simulink library "Library_ASK"  (R2018b)
settings: Solver=VariableStepAuto  StartTime=0.0  StopTime=10.0  RelTol=1e-3  EnableMultiTasking=on
undefined symbols (not defined in the file): akt_2GTR_az_HA, akt_2GTR_az_VA, akt_2GTR_rn_HA, akt_2GTR_rn_VA, akt_GTR_az_HA, akt_GTR_az_VA, akt_GTR_rn_HA, akt_GTR_rn_VA, alpha, b_zahn, beta_b, breakpointset, choose_ulg, DiscIntNeverNeededParam, eps_1, eps_2, eps_alpha, eta_aa, eta_Kegel_max, Fx_LSD_max, Fx_mUELG_max, i_DF, i_Kegelrad_OD, i_TRM_G1_HA, i_TRM_G1_VA, i_TRM_G2_HA, i_TRM_G2_VA, i_TRM_HA, i_TRM_Stufe_1_HA, i_TRM_Stufe_1_VA, i_TRM_Stufe_2_HA, i_TRM_Stufe_2_VA, i_TRM_VA, M_Cl_LSD_max, M_Cl_mUELG_max, M_EM_max, M_Kupplung_mUELG_Schlepp, mu_cl_LSD, mu_cl_mUELG, n_EM_max, n_Stufen_TRM_HA, n_Stufen_TRM_VA, ndyn_oil, nreib_LSD, nreib_mUELG, par_MDT, par_VEH, Ra, rm_LSD, rm_mUELG, select_Traktion_split, stepsize, wkg_Diff_mUELG, wkg_GTR, X_L, z_atts, z_ayc, z_ayc_lr, z_ayc_rl
libraries: simulink x23, $bdroot x6
(part 1 of 4)
settings Model: Creator=ga25fis  LastModifiedBy=ga35gug
settings DataIOCC: LimitDataPoints=on
settings OptimizationCC: LifeSpan=inf
settings DebuggingCC: AllowSymbolicDim=off  SFUnexpectedBacktrackingDiag=warning  SFNoUnconditionalDefaultTransitionDiag=warning  SFExecutionAtInitializationDiag=none
settings ModelReferenceCC: PropagateSignalLabelsOutOfModel=off
settings SFSimCC: SimUseLocalCustomCode=off
settings RTWCC: RTWUseLocalCustomCode=off
settings CodeAppCC: StateflowObjectComments=on
settings GRTTargetCC: TargetLangStandard=C89/C90 (ANSI)
settings ConfigComp: CovMetricSettings=dw  CovHtmlReporting=on  CovSaveCumulativeToWorkspaceVar=on  CovSaveSingleToWorkspaceVar=on  CovExternalEMLEnable=off

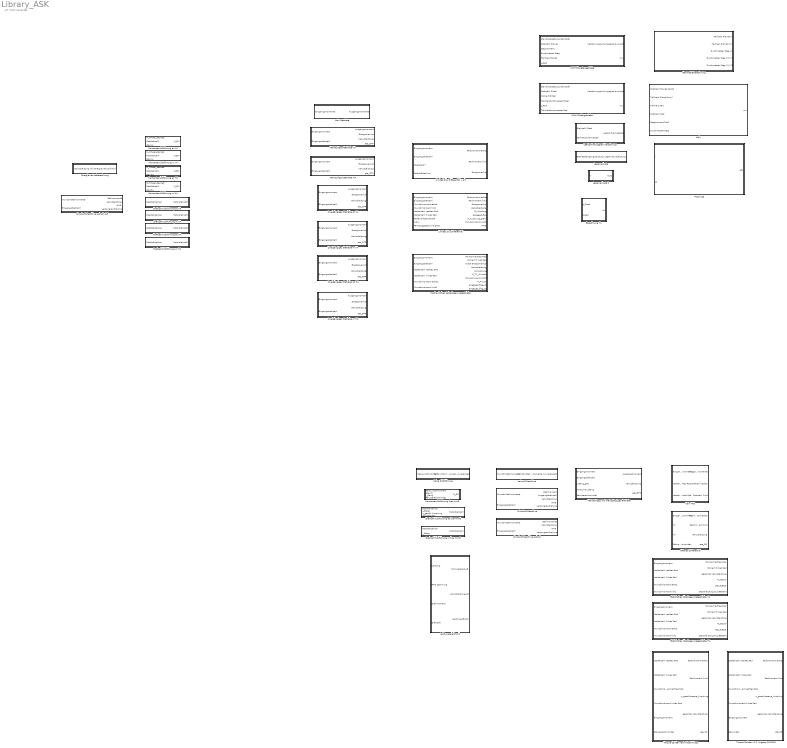
== system Library_ASK ==
  note: ALT / Nicht verwendet
  Berechnung Hv : Subsystem
  Drehzahlrückführung az HA : Subsystem
      mask Display: set_param(gcb, 'BackgroundColor', '[0.9,0.7,1]');
  Drehzahlrückführung az VA : Subsystem
      mask Display: set_param(gcb, 'BackgroundColor', '[0.9,0.7,1]');
  Drehzahlrückführung az fuer mmG : Subsystem
      mask Display: set_param(gcb, 'BackgroundColor', '[0.9,0.7,1]');
  Drehzahlrückführung rn HA : Subsystem
      mask Display: set_param(gcb, 'BackgroundColor', '[0.9,0.7,1]');
  Drehzahlrückführung rn VA : Subsystem
      mask Display: set_param(gcb, 'BackgroundColor', '[0.9,0.7,1]');
  Drehzahlrückführung rn fuer mmG : Subsystem
      mask Display: set_param(gcb, 'BackgroundColor', '[0.9,0.7,1]');
  Elektrisches Überlagerungsgetriebe HA : Subsystem
      settings: MinAlgLoopOccurrences=on
      mask Display: set_param(gcb, 'BackgroundColor', '[0,1,0.6]');
  Elektrisches Überlagerungsgetriebe VA : Subsystem
      settings: MinAlgLoopOccurrences=on
      mask Display: set_param(gcb, 'BackgroundColor', '[0,1,0.6]');
  Energieverlustberechnung : Subsystem
      mask Display: set_param(gcb, 'BackgroundColor', '[0.3,0.3,0.6]');
  Geometrieberechnung : Subsystem
  Kein Getriebe : Subsystem
      settings: MinAlgLoopOccurrences=on
      mask Display: set_param(gcb, 'BackgroundColor', '[0.9,0.1,0.4]');
  Kein MVS : Subsystem
      mask Display: set_param(gcb, 'BackgroundColor', '[0,1,0.6]');
  Keine E-Maschine : Subsystem
      settings: MinAlgLoopOccurrences=on
      mask Display: set_param(gcb, 'BackgroundColor', '[0.5,0.7,1]');
  Keine Rückführung : Subsystem
      mask Display: set_param(gcb, 'BackgroundColor', '[0.9,0.7,1]');
  Kelly : Subsystem
  Lagerverluste : Subsystem
  Lagerverluste 2 : Subsystem
  Leerlaufverlustgrad Verzahnung : Subsystem
  Leistungselektronik : Subsystem  mask{Efficiency_Map=0, Current=0, Voltage=0, Powerfactor=0, Powerfactor_Map=0, Torque=0, Speed=0}
      mask prompts: Current "Strom"; Voltage "Spannung"; Torque "Drehmoment"; Speed "Drehzahl"
      mask DialogControl ParameterGroupVar Prompt: Efficiency_Map
      mask DialogControl ParameterGroupVar_copy Prompt: Powerfactor_Map
  Limited Slip Differential : Subsystem
      settings: MinAlgLoopOccurrences=on
      mask Display: set_param(gcb, 'BackgroundColor', '[0,1,0.6]');
  "Limited Slip Differential -- alt" : Subsystem
      settings: MinAlgLoopOccurrences=on
      mask Display: set_param(gcb, 'BackgroundColor', '[0,1,0.6]');
  Mehrstufiges Getriebe HA : Subsystem
      settings: MinAlgLoopOccurrences=on
      mask Display: set_param(gcb, 'BackgroundColor', '[0.9,0.1,0.4]');
  Mehrstufiges Getriebe VA : Subsystem
      settings: MinAlgLoopOccurrences=on
      mask Display: set_param(gcb, 'BackgroundColor', '[0.9,0.1,0.4]');
  Mehrstufiges und mehrgängiges Getriebe : Subsystem
      settings: MinAlgLoopOccurrences=on
      mask Display: set_param(gcb, 'BackgroundColor', '[0.9,0.1,0.4]');
  Momentenrückführung az HA : Subsystem
      mask Display: set_param(gcb, 'BackgroundColor', '[0.9,0.7,1]');
  Momentenrückführung az VA : Subsystem
      mask Display: set_param(gcb, 'BackgroundColor', '[0.9,0.7,1]');
  Momentenrückführung fuer mmG : Subsystem
      mask Display: set_param(gcb, 'BackgroundColor', '[0.9,0.7,1]');
  Momentenrückführung rn HA : Subsystem
      mask Display: set_param(gcb, 'BackgroundColor', '[0.9,0.7,1]');
  Momentenrückführung rn VA : Subsystem
      mask Display: set_param(gcb, 'BackgroundColor', '[0.9,0.7,1]');
  NWH Planetengetriebe : Subsystem
      mask Display: set_param(gcb, 'BackgroundColor', '[0.8,0.8,0.8]');
  NWH Stufengetriebe : Subsystem
      mask Display: set_param(gcb, 'BackgroundColor', '[0.8,0.8,0.8]');
  Offenes Differential : Subsystem  mask{M_max=par_MDT.VA.em.M_max_mot, i_max=par_MDT.VA.trans.imax}
      settings: MinAlgLoopOccurrences=on
      mask Display: set_param(gcb, 'BackgroundColor', '[0,1,0.6]');
  Poppinga : Subsystem
  Simple E-Maschine : Subsystem  mask{Mot_Mmax_Curve=par_MDT.VA.em.MaxMotorTrqCurve_M, Mot_nmax_Curve=par_MDT.VA.em.MaxMotorTrqCurve_w, Gen_Mmax_Curve=par_MDT.VA.em.MaxGeneratorTrqCurve_M, Gen_nmax_Curve=par_MDT.VA.em.MaxGeneratorTrqCurve_w, Mot_Pesce_Mat=par_MDT.VA.em.MotorEffMap3D, Mot_Pesce_y=par_MDT.VA.em.MotorEffMap3D_w, Mot_Pesce_z=par_MDT.VA.em.MotorEffMap3D_M, Gen_Pesce_Mat=par_MDT.VA.em.GeneratorEffMap3D, Gen_Pesce_y=par_MDT.VA.em.GeneratorEffMap3D_w, Gen_Pesce_z=par_MDT.VA.em.GeneratorEffMap3D_M}
      settings: MinAlgLoopOccurrences=on
      mask Display: set_param(gcb, 'BackgroundColor', '[0.5,0.7,1]');
  Simple E-Maschine radnah : Subsystem  mask{Mot_Mmax_Curve=par_MDT.VA.em.MaxMotorTrqCurve_M, Mot_nmax_Curve=par_MDT.VA.em.MaxMotorTrqCurve_w, Gen_Mmax_Curve=par_MDT.VA.em.MaxGeneratorTrqCurve_M, Gen_nmax_Curve=par_MDT.VA.em.MaxGeneratorTrqCurve_w, Mot_Pesce_Mat=par_MDT.VA.em.MotorEffMap3D, Mot_Pesce_y=par_MDT.VA.em.MotorEffMap3D_w, Mot_Pesce_z=par_MDT.VA.em.MotorEffMap3D_M, Gen_Pesce_Mat=par_MDT.VA.em.GeneratorEffMap3D, Gen_Pesce_y=par_MDT.VA.em.GeneratorEffMap3D_w, Gen_Pesce_z=par_MDT.VA.em.GeneratorEffMap3D_M}
      settings: MinAlgLoopOccurrences=on
      mask Display: set_param(gcb, 'BackgroundColor', '[0.5,0.7,1]');
  Simple E-Maschine radnah ALT : Subsystem  mask{Mot_Mmax_Curve=par_VEH.dt.em.MmaxCurve_mot_VA, Mot_nmax_Curve=par_VEH.dt.em.nmaxCurve_mot_VA, Gen_Mmax_Curve=par_VEH.dt.em.MmaxCurve_gen_VA, Gen_nmax_Curve=par_VEH.dt.em.nmaxCurve_gen_VA, Mot_Pesce_Mat=par_VEH.dt.em.EffMapData_mot_VA, Mot_Pesce_y=par_VEH.dt.em.MotorEffMap3D_y_VA, Mot_Pesce_z=par_VEH.dt.em.MotorEffMap3D_z_VA, Gen_Pesce_Mat=par_VEH.dt.em.EffMapData_gen_VA, Gen_Pesce_y=par_VEH.dt.em.GeneratorEffMap3D_y_VA, Gen_Pesce_z=par_VEH.dt.em.GeneratorEffMap3D_z_VA}
      settings: MinAlgLoopOccurrences=on
      mask Display: set_param(gcb, 'BackgroundColor', '[0.5,0.7,1]');
  Torque Splitter nach Arbeit Tripps : Subsystem  TreatAsAtomicUnit=on
  Torque Splitter v2 C. Angerer 10/2018 : Subsystem
  Zweigängiges Getriebe az HA : Subsystem
      mask Display: set_param(gcb, 'BackgroundColor', '[0.9,0.1,0.4]');
  Zweigängiges Getriebe az VA : Subsystem
      mask Display: set_param(gcb, 'BackgroundColor', '[0.9,0.1,0.4]');
  Zweigängiges Getriebe rn HA : Subsystem
      mask Display: set_param(gcb, 'BackgroundColor', '[0.9,0.1,0.4]');
  Zweigängiges Getriebe rn VA : Subsystem
      mask Display: set_param(gcb, 'BackgroundColor', '[0.9,0.1,0.4]');
  mechanisches Ueberlagerungsgetriebe : Subsystem
      settings: MinAlgLoopOccurrences=on
      mask Display: set_param(gcb, 'BackgroundColor', '[0,1,0.6]');

== system Library_ASK/Berechnung Hv ==
  note: wegen Hohlrad
  z_Ritzel : Inport
  z_Rad : Inport  Port=2
  Abs : Abs
  Add : Sum
  Add1 : Sum  Inputs=+-++
  Berechnung i : Product  Inputs=*/
  Constant : Constant
  Constant1 : Constant
  Divide : Product  Inputs=*///
  Gain : Gain  Gain=pi
  Grundkreisschrägungswinkel : Constant  Value=par_VEH.trans.beta_b
  Kopfüberdeckung Rad : Constant  Value=par_VEH.trans.eps_2
  Kopfüberdeckung Ritzel : Constant  Value=par_VEH.trans.eps_1
  Math Function : Math  Operator=square  SaturateOnIntegerOverflow=on
  Math Function1 : Math  Operator=square  SaturateOnIntegerOverflow=on
  Product : Product
  Profilüberdeckung : Constant  Value=par_VEH.trans.alpha
  Trigonometric Function : Trigonometry  Operator=cos
  Hv : Outport
  wires:
  z_Ritzel/1 -> Divide/3, Berechnung i/2
  z_Rad/1 -> Abs/1
  Constant1/1 -> Add/1
  Berechnung i/1 -> Divide/2, Add/2
  Add/1 -> Gain/1
  Grundkreisschrägungswinkel/1 -> Trigonometric Function/1
  Gain/1 -> Divide/1
  Trigonometric Function/1 -> Divide/4
  Divide/1 -> Product/1
  Kopfüberdeckung Ritzel/1 -> Math Function/1
  Math Function/1 -> Add1/3
  Math Function1/1 -> Add1/4
  Kopfüberdeckung Rad/1 -> Math Function1/1
  Profilüberdeckung/1 -> Add1/2
  Constant/1 -> Add1/1
  Add1/1 -> Product/2
  Product/1 -> Hv/1
  Abs/1 -> Berechnung i/1

== system Library_ASK/Drehzahlrückführung az HA ==
  note: Das hier ist nur für die az gedacht! Die radnahen kriegen ihre Drehzahlen von den MVS über die from - Blöcke
  Raddrehzahlen : Inport
  Add : Sum
  Constant : Constant  Value=akt_GTR_az_HA
  Constant1 : Constant  Value=akt_2GTR_az_HA
  Demux : Demux  Outputs=2
  Fall Einganggetriebe : Subsystem
  Fall Zweiganggetriebe : Subsystem
  Gain : Gain  Gain=0.5
  Switch : Switch  Criteria=u2 > Threshold
  Motordrehzahl : Outport
  wires:
  Constant1/1 -> Fall Zweiganggetriebe/Enable
  Constant/1 -> Fall Einganggetriebe/Enable, Switch/2
  Fall Einganggetriebe/1(Motordrehzahl) -> Switch/1
  Switch/1 -> Motordrehzahl/1
  Fall Zweiganggetriebe/1(Motordrehzahl) -> Switch/3
  Gain/1 -> Fall Zweiganggetriebe/1(Mittlere Raddrehzahl), Fall Einganggetriebe/1(Mittlere Raddrehzahl)
  Raddrehzahlen/1 -> Demux/1
  Demux/1 -> Add/1
  Demux/2 -> Add/2
  Add/1 -> Gain/1

== system Library_ASK/Drehzahlrückführung az VA ==
  note: Das hier ist nur für die az gedacht! Die radnahen kriegen ihre Drehzahlen von den MVS über die from - Blöcke
  Raddrehzahlen : Inport
  Add : Sum
  Constant : Constant  Value=akt_GTR_az_VA
  Constant1 : Constant  Value=akt_2GTR_az_VA
  Demux : Demux  Outputs=2
  Fall Einganggetriebe : Subsystem
  Fall Zweiganggetriebe : Subsystem
  Gain : Gain  Gain=0.5
  Switch : Switch  Criteria=u2 > Threshold
  Motordrehzahl : Outport
  wires:
  Add/1 -> Gain/1
  Demux/2 -> Add/2
  Demux/1 -> Add/1
  Raddrehzahlen/1 -> Demux/1
  Gain/1 -> Fall Einganggetriebe/1(Mittlere Raddrehzahl), Fall Zweiganggetriebe/1(Mittlere Raddrehzahl)
  Fall Zweiganggetriebe/1(Motordrehzahl) -> Switch/3
  Switch/1 -> Motordrehzahl/1
  Fall Einganggetriebe/1(Motordrehzahl) -> Switch/1
  Constant/1 -> Switch/2, Fall Einganggetriebe/Enable
  Constant1/1 -> Fall Zweiganggetriebe/Enable

== system Library_ASK/Drehzahlrückführung az fuer mmG ==
  note: Das hier ist nur für die az gedacht! Die radnahen kriegen ihre Drehzahlen von den MVS über die from - Blöcke
  Raddrehzahlen : Inport
  i_Gang : Inport  Port=2
  n_geschl Kupplung : Inport  Port=3
  Aktivator TS : Inport  Port=4
  Enable : EnablePort
  Add11 : Sum
  Demux : Demux  Outputs=2
  Divide4 : Product  Inputs=**
  Gain : Gain  Gain=0.5
  Switch : Switch  Criteria=u2 > Threshold
  Motordrehzahl : Outport
  wires:
  Demux/2 -> Add11/2
  Gain/1 -> Switch/3
  Add11/1 -> Gain/1
  Switch/1 -> Divide4/1
  n_geschl Kupplung/1 -> Switch/1
  Divide4/1 -> Motordrehzahl/1
  Aktivator TS/1 -> Switch/2
  i_Gang/1 -> Divide4/2
  Raddrehzahlen/1 -> Demux/1
  Demux/1 -> Add11/1

== system Library_ASK/Drehzahlrückführung rn HA ==
  Raddrehzahlen : Inport
  Constant : Constant  Value=akt_GTR_rn_HA
  Constant1 : Constant  Value=akt_2GTR_rn_HA
  Fall Einganggetriebe : Subsystem
  Fall Zweiganggetriebe : Subsystem
  Switch : Switch  Criteria=u2 > Threshold
  Motordrehzahl : Outport
  wires:
  Raddrehzahlen/1 -> Fall Einganggetriebe/1(Mittlere Raddrehzahl), Fall Zweiganggetriebe/1(Raddrehzahl)
  Fall Zweiganggetriebe/1(Motordrehzahl) -> Switch/3
  Switch/1 -> Motordrehzahl/1
  Fall Einganggetriebe/1(Motordrehzahl) -> Switch/1
  Constant/1 -> Switch/2, Fall Einganggetriebe/Enable
  Constant1/1 -> Fall Zweiganggetriebe/Enable

== system Library_ASK/Drehzahlrückführung rn VA ==
  Raddrehzahlen : Inport
  Constant : Constant  Value=akt_GTR_rn_VA
  Constant1 : Constant  Value=akt_2GTR_rn_VA
  Fall Einganggetriebe : Subsystem
  Fall Zweiganggetriebe : Subsystem
  Switch : Switch  Criteria=u2 > Threshold
  Motordrehzahl : Outport
  wires:
  Constant1/1 -> Fall Zweiganggetriebe/Enable
  Constant/1 -> Fall Einganggetriebe/Enable, Switch/2
  Fall Einganggetriebe/1(Motordrehzahl) -> Switch/1
  Switch/1 -> Motordrehzahl/1
  Fall Zweiganggetriebe/1(Motordrehzahl) -> Switch/3
  Raddrehzahlen/1 -> Fall Zweiganggetriebe/1(Raddrehzahl), Fall Einganggetriebe/1(Raddrehzahl)

== system Library_ASK/Drehzahlrückführung rn fuer mmG ==
  Raddrehzahlen : Inport
  i_Gang : Inport  Port=2
  Enable : EnablePort
  Divide : Product  Inputs=**
  Motordrehzahl : Outport
  wires:
  i_Gang/1 -> Divide/2
  Raddrehzahlen/1 -> Divide/1
  Divide/1 -> Motordrehzahl/1

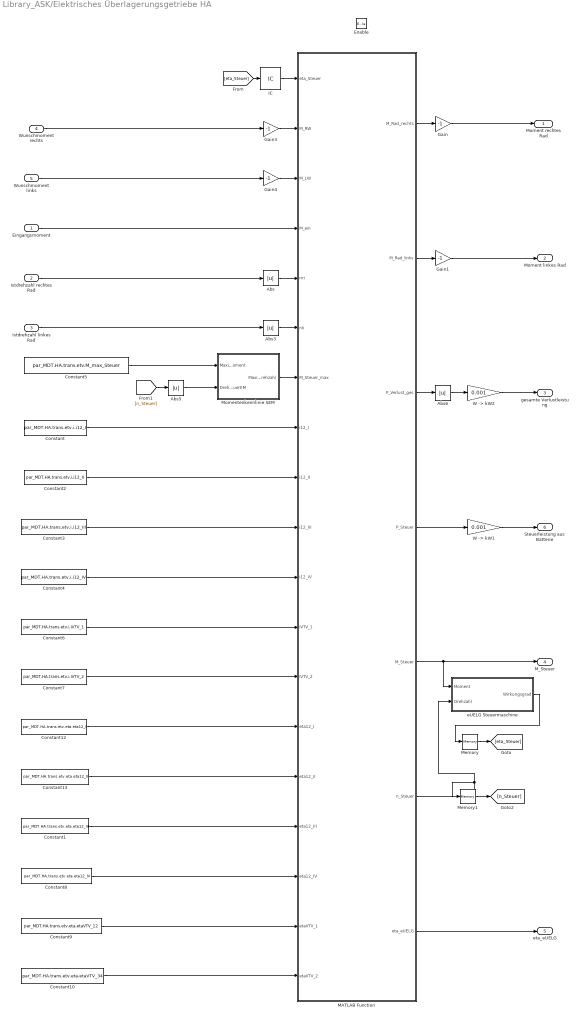
== system Library_ASK/Elektrisches Überlagerungsgetriebe HA ==
  Eingangsmoment : Inport
  Istdrehzahl rechtes Rad : Inport  Port=2
  Istdrehzahl linkes Rad : Inport  Port=3
  Wunschmoment rechts : Inport  Port=4
  Wunschmoment links : Inport  Port=5
  Enable : EnablePort
  Abs{,3,5..6} (4 alike) : Abs
  Constant : Constant  Value=par_MDT.HA.trans.etv.i.i12_I
  Constant1 : Constant  Value=par_MDT.HA.trans.etv.eta.eta12_III
  Constant10 : Constant  Value=par_MDT.HA.trans.etv.eta.etaVTV_34
  Constant12 : Constant  Value=par_MDT.HA.trans.etv.eta.eta12_I
  Constant13 : Constant  Value=par_MDT.HA.trans.etv.eta.eta12_II
  Constant2 : Constant  Value=par_MDT.HA.trans.etv.i.i12_II
  Constant3 : Constant  Value=par_MDT.HA.trans.etv.i.i12_III
  Constant4 : Constant  Value=par_MDT.HA.trans.etv.i.i12_IV
  Constant5 : Constant  Value=par_MDT.HA.trans.etv.M_max_Steuer
  Constant6 : Constant  Value=par_MDT.HA.trans.etv.i.iVTV_1
  Constant7 : Constant  Value=par_MDT.HA.trans.etv.i.iVTV_2
  Constant8 : Constant  Value=par_MDT.HA.trans.etv.eta.eta12_IV
  Constant9 : Constant  Value=par_MDT.HA.trans.etv.eta.etaVTV_12
  Gain{,1,3..4} (4 alike) : Gain  Gain=-1
  IC : InitialCondition  Value=0.5
  MATLAB Function : MATLAB Function  TreatAsAtomicUnit=on
  Memory : Memory
  Memory1 : Memory
  Momentenkennlinie SEM : Subsystem
  "W -> kW1" : Gain  Gain=0.001
  "W -> kW2" : Gain  Gain=0.001
  eUELG Steuermaschine : Subsystem
      settings: MinAlgLoopOccurrences=on
      mask Display: set_param(gcb, 'BackgroundColor', '[0.5,0.7,1]');
  Moment rechtes Rad : Outport  InitialOutput=0
  Moment linkes Rad : Outport  Port=2  InitialOutput=0
  gesamte Verlustleistung : Outport  Port=3  InitialOutput=0
  M_Steuer : Outport  Port=4
  eta_eUELG : Outport  Port=5
  Steuerleistung aus Batterie : Outport  Port=6
  wires:
  Abs6/1 -> "W -> kW2"/1
  MATLAB Function/4(P_Steuer) -> "W -> kW1"/1
  "W -> kW1"/1 -> Steuerleistung aus Batterie/1
  Gain4/1 -> MATLAB Function/3(M_LW)
  Gain3/1 -> MATLAB Function/2(M_RW)
  Constant8/1 -> MATLAB Function/17(eta12_IV)
  Istdrehzahl linkes Rad/1 -> Abs3/1
  Istdrehzahl rechtes Rad/1 -> Abs/1
  Constant10/1 -> MATLAB Function/19(etaVTV_2)
  Constant9/1 -> MATLAB Function/18(etaVTV_1)
  Constant1/1 -> MATLAB Function/16(eta12_III)
  Wunschmoment links/1 -> Gain4/1
  Wunschmoment rechts/1 -> Gain3/1
  Gain1/1 -> Moment linkes Rad/1
  Gain/1 -> Moment rechtes Rad/1
  Abs5/1 -> Momentenkennlinie SEM/2(Drehzahl SteuerEM)
  Memory1/1 -> [n_Steuer]
  [n_Steuer] -> Abs5/1
  Momentenkennlinie SEM/1(Maximalmoment bei Drehzahl) -> MATLAB Function/7(M_Steuer_max)
  Constant5/1 -> Momentenkennlinie SEM/1(Maximalmoment)
  Abs3/1 -> MATLAB Function/6(nli)
  Abs/1 -> MATLAB Function/5(nri)
  Constant7/1 -> MATLAB Function/13(iVTV_2)
  Constant6/1 -> MATLAB Function/12(iVTV_1)
  MATLAB Function/7(eta_eUELG) -> eta_eUELG/1
  Eingangsmoment/1 -> MATLAB Function/4(M_ein)
  MATLAB Function/5(M_Steuer) -> eUELG Steuermaschine/1(Moment), M_Steuer/1
  "W -> kW2"/1 -> gesamte Verlustleistung/1
  MATLAB Function/6(n_Steuer) -> Memory1/1, eUELG Steuermaschine/2(Drehzahl)
  Constant13/1 -> MATLAB Function/15(eta12_II)
  Constant12/1 -> MATLAB Function/14(eta12_I)
  Constant4/1 -> MATLAB Function/11(i12_IV)
  Constant3/1 -> MATLAB Function/10(i12_III)
  Constant2/1 -> MATLAB Function/9(i12_II)
  Constant/1 -> MATLAB Function/8(i12_I)
  IC/1 -> MATLAB Function/1(eta_Steuer)
  Memory/1 -> [eta_Steuer]
  eUELG Steuermaschine/1(Wirkungsgrad) -> Memory/1
  [eta_Steuer] -> IC/1
  MATLAB Function/3(P_Verlust_ges) -> Abs6/1
  MATLAB Function/2(M_Rad_links) -> Gain1/1
  MATLAB Function/1(M_Rad_rechts) -> Gain/1

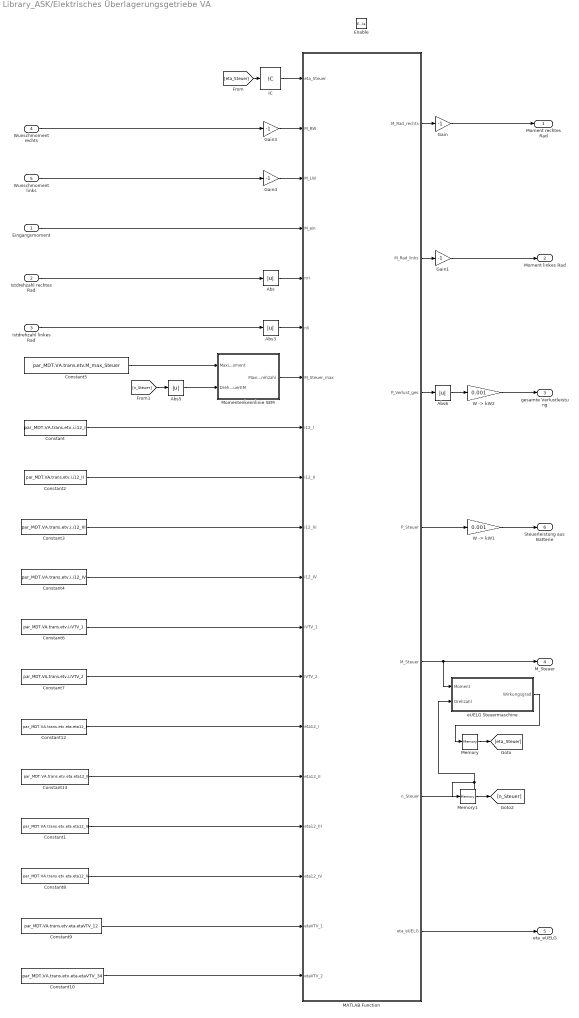
== system Library_ASK/Elektrisches Überlagerungsgetriebe VA ==
  Eingangsmoment : Inport
  Istdrehzahl rechtes Rad : Inport  Port=2
  Istdrehzahl linkes Rad : Inport  Port=3
  Wunschmoment rechts : Inport  Port=4
  Wunschmoment links : Inport  Port=5
  Enable : EnablePort
  Abs{,3,5..6} (4 alike) : Abs
  Constant : Constant  Value=par_MDT.VA.trans.etv.i.i12_I
  Constant1 : Constant  Value=par_MDT.VA.trans.etv.eta.eta12_III
  Constant10 : Constant  Value=par_MDT.VA.trans.etv.eta.etaVTV_34
  Constant12 : Constant  Value=par_MDT.VA.trans.etv.eta.eta12_I
  Constant13 : Constant  Value=par_MDT.VA.trans.etv.eta.eta12_II
  Constant2 : Constant  Value=par_MDT.VA.trans.etv.i.i12_II
  Constant3 : Constant  Value=par_MDT.VA.trans.etv.i.i12_III
  Constant4 : Constant  Value=par_MDT.VA.trans.etv.i.i12_IV
  Constant5 : Constant  Value=par_MDT.VA.trans.etv.M_max_Steuer
  Constant6 : Constant  Value=par_MDT.VA.trans.etv.i.iVTV_1
  Constant7 : Constant  Value=par_MDT.VA.trans.etv.i.iVTV_2
  Constant8 : Constant  Value=par_MDT.VA.trans.etv.eta.eta12_IV
  Constant9 : Constant  Value=par_MDT.VA.trans.etv.eta.etaVTV_12
  Gain{,1,3..4} (4 alike) : Gain  Gain=-1
  IC : InitialCondition  Value=0.5
  MATLAB Function : MATLAB Function  TreatAsAtomicUnit=on
  Memory : Memory
  Memory1 : Memory
  Momentenkennlinie SEM : Subsystem
  "W -> kW1" : Gain  Gain=0.001
  "W -> kW2" : Gain  Gain=0.001
  eUELG Steuermaschine : Subsystem
      settings: MinAlgLoopOccurrences=on
  Moment rechtes Rad : Outport  InitialOutput=0
  Moment linkes Rad : Outport  Port=2  InitialOutput=0
  gesamte Verlustleistung : Outport  Port=3  InitialOutput=0
  M_Steuer : Outport  Port=4
  eta_eUELG : Outport  Port=5
  Steuerleistung aus Batterie : Outport  Port=6
  wires:
  MATLAB Function/1(M_Rad_rechts) -> Gain/1
  MATLAB Function/2(M_Rad_links) -> Gain1/1
  MATLAB Function/3(P_Verlust_ges) -> Abs6/1
  [eta_Steuer] -> IC/1
  eUELG Steuermaschine/1(Wirkungsgrad) -> Memory/1
  Memory/1 -> [eta_Steuer]
  IC/1 -> MATLAB Function/1(eta_Steuer)
  Constant/1 -> MATLAB Function/8(i12_I)
  Constant2/1 -> MATLAB Function/9(i12_II)
  Constant3/1 -> MATLAB Function/10(i12_III)
  Constant4/1 -> MATLAB Function/11(i12_IV)
  Constant12/1 -> MATLAB Function/14(eta12_I)
  Constant13/1 -> MATLAB Function/15(eta12_II)
  MATLAB Function/6(n_Steuer) -> eUELG Steuermaschine/2(Drehzahl), Memory1/1
  "W -> kW2"/1 -> gesamte Verlustleistung/1
  MATLAB Function/5(M_Steuer) -> M_Steuer/1, eUELG Steuermaschine/1(Moment)
  Eingangsmoment/1 -> MATLAB Function/4(M_ein)
  MATLAB Function/7(eta_eUELG) -> eta_eUELG/1
  Constant6/1 -> MATLAB Function/12(iVTV_1)
  Constant7/1 -> MATLAB Function/13(iVTV_2)
  Abs/1 -> MATLAB Function/5(nri)
  Abs3/1 -> MATLAB Function/6(nli)
  Constant5/1 -> Momentenkennlinie SEM/1(Maximalmoment)
  Momentenkennlinie SEM/1(Maximalmoment bei Drehzahl) -> MATLAB Function/7(M_Steuer_max)
  [n_Steuer] -> Abs5/1
  Memory1/1 -> [n_Steuer]
  Abs5/1 -> Momentenkennlinie SEM/2(Drehzahl SteuerEM)
  Gain/1 -> Moment rechtes Rad/1
  Gain1/1 -> Moment linkes Rad/1
  Wunschmoment rechts/1 -> Gain3/1
  Wunschmoment links/1 -> Gain4/1
  Constant1/1 -> MATLAB Function/16(eta12_III)
  Constant9/1 -> MATLAB Function/18(etaVTV_1)
  Constant10/1 -> MATLAB Function/19(etaVTV_2)
  Istdrehzahl rechtes Rad/1 -> Abs/1
  Istdrehzahl linkes Rad/1 -> Abs3/1
  Constant8/1 -> MATLAB Function/17(eta12_IV)
  Gain3/1 -> MATLAB Function/2(M_RW)
  Gain4/1 -> MATLAB Function/3(M_LW)
  "W -> kW1"/1 -> Steuerleistung aus Batterie/1
  MATLAB Function/4(P_Steuer) -> "W -> kW1"/1
  Abs6/1 -> "W -> kW2"/1

== system Library_ASK/Energieverlustberechnung ==
  Verlustleistung [W] : Inport
  Abs : Abs
  Discrete-Time Integrator : DiscreteIntegrator  gainval=1  SampleTime=-1  ICPrevOutput=DiscIntNeverNeededParam  ICPrevScaledInput=DiscIntNeverNeededParam
  "Ws -> kWh" : Gain  Gain=1/3600000
  Energieverlust [kWh] : Outport
  wires:
  Verlustleistung [W]/1 -> Abs/1
  Discrete-Time Integrator/1 -> "Ws -> kWh"/1
  "Ws -> kWh"/1 -> Energieverlust [kWh]/1
  Abs/1 -> Discrete-Time Integrator/1

== system Library_ASK/Geometrieberechnung ==
  note: Die eine Zähnezahl sitzt nach der einmaligen Initialisierung im Workspace und kommt hier als constant rein,
      | die andere kommt aus dem par_VEH und deshalb als input. Sie ist eine Benutzervorgabe bzw, Variierungsgröße.
  Add : Sum
  Add1 : Sum
  Add2 : Sum
  Modul I/II : Constant
  Modul III/IV : Constant  Value=1.85
  Product{,1..4} (5 alike) : Product
  z1_I : Constant  Value=41
  z1_III : Constant  Value=36
  z2_III : Constant  Value=39
  zP_III_IV : Constant  Value=15
  zP_I_II : Constant  Value=23
  Teilkreis Planet I/II : Outport
  Teilkreis Planet III/IV : Outport  Port=2
  Durchmesser Steg I/II : Outport  Port=3
  Durchmesser Steg III/IV 1 : Outport  Port=4
  Durchmesser Steg III/IV 2 : Outport  Port=5
  wires:
  Product/1 -> Teilkreis Planet I/II/1
  Modul I/II/1 -> Product1/1, Product/1
  zP_I_II/1 -> Add/2, Product/2
  Product2/1 -> Teilkreis Planet III/IV/1
  Modul III/IV/1 -> Product4/1, Product3/1, Product2/1
  zP_III_IV/1 -> Add2/2, Add1/2, Product2/2
  z1_I/1 -> Add/1
  Add/1 -> Product1/2
  Product1/1 -> Durchmesser Steg I/II/1
  z2_III/1 -> Add1/1
  Add1/1 -> Product3/2
  Product3/1 -> Durchmesser Steg III/IV 1/1
  z1_III/1 -> Add2/1
  Add2/1 -> Product4/2
  Product4/1 -> Durchmesser Steg III/IV 2/1

== system Library_ASK/Kein Getriebe ==
  Eingangsmomente : Inport
  Enable : EnablePort
  Ausgangsmomente : Outport  InitialOutput=0
  wires:
  Eingangsmomente/1 -> Ausgangsmomente/1

== system Library_ASK/Kein MVS ==
  Eingangsmomente : Inport
  Istdrehzahl rechtes Rad : Inport  Port=2
  Istdrehzahl linkes Rad : Inport  Port=3
  Enable : EnablePort
  Ausgangsmomente : Outport  InitialOutput=0
  Drehzahl rechts : Outport  Port=2  InitialOutput=0
  Drehzahl links : Outport  Port=3  InitialOutput=0
  wires:
  Istdrehzahl linkes Rad/1 -> Drehzahl links/1
  Istdrehzahl rechtes Rad/1 -> Drehzahl rechts/1
  Eingangsmomente/1 -> Ausgangsmomente/1

== system Library_ASK/Keine E-Maschine ==
  Wunsch-Stellmomente : Inport
  Enable : EnablePort
  Wunsch-Stellmomente (unverändert) : Outport  InitialOutput=0
  wires:
  Wunsch-Stellmomente/1 -> Wunsch-Stellmomente (unverändert)/1

== system Library_ASK/Keine Rückführung ==
  Radwunschmoment : Inport
  Enable : EnablePort
  Radwunschmoment unverändert : Outport
  wires:
  Radwunschmoment/1 -> Radwunschmoment unverändert/1

== system Library_ASK/Kelly ==
  Drehzahl Planet [rad/s] : Inport
  Teilkreis Planet [mm] : Inport  Port=2
  Teilkreis Rad : Inport  Port=3
  Drehzahl Rad : Inport  Port=4
  Stegmoment [Nm] : Inport  Port=5
  Durchmesser Steg : Inport  Port=6
  Abs : Abs
  Abs1 : Abs
  Add : Sum  Inputs=+-
  Constant : Constant  Value=alpha
  Constant2 : Constant  Value=317000000
  Divide : Product  Inputs=***
  Divide3 : Product  Inputs=*/
  Gain : Gain  Gain=0.5
  Gain1 : Gain  Gain=0.5
  Gain3 : Gain  Gain=0.0127
  Math Function : Math  Operator=log10  SaturateOnIntegerOverflow=on
  Product : Product
  Product1 : Product
  Sliding speed : Product
  Trigonometric Function : Trigonometry
  "m/s -> in/s" : Gain  Gain=39.37
  "m/s -> in/s1" : Gain  Gain=39.37
  "mm/s -> m/s" : Gain  Gain=0.001
  x-Achsen-Parameter : Subsystem
  mu : Outport
  wires:
  Teilkreis Planet [mm]/1 -> Gain/1
  Teilkreis Rad/1 -> Gain1/1
  Drehzahl Planet [rad/s]/1 -> x-Achsen-Parameter/1(Drehzahl Planet), Product/1
  Gain1/1 -> Product1/1
  Drehzahl Rad/1 -> Product1/2
  Product/1 -> Add/1
  Product1/1 -> Add/2
  Add/1 -> "mm/s -> m/s"/1
  Constant/1 -> Trigonometric Function/1
  Trigonometric Function/1 -> Sliding speed/1
  Gain/1 -> x-Achsen-Parameter/2(Teilkreis Planet), Product/2
  Sliding speed/1 -> Abs/1
  Divide/1 -> Divide3/2
  Constant2/1 -> Divide3/1
  Divide3/1 -> Math Function/1
  Math Function/1 -> Gain3/1
  Gain3/1 -> mu/1
  Stegmoment [Nm]/1 -> x-Achsen-Parameter/3(Stegmoment)
  Durchmesser Steg/1 -> x-Achsen-Parameter/4(Durchmesser Steg)
  x-Achsen-Parameter/1(mu0*vs/W) -> Abs1/1
  Abs/1 -> "m/s -> in/s1"/1, "m/s -> in/s"/1
  "m/s -> in/s"/1 -> Divide/1
  "m/s -> in/s1"/1 -> Divide/2
  "mm/s -> m/s"/1 -> Sliding speed/2
  Abs1/1 -> Divide/3

== system Library_ASK/Lagerverluste ==
  Getriebeeingangsleistung : Inport
  Gain : Gain  Gain=0.001
  Lagerverlustleistung : Outport
  wires:
  Getriebeeingangsleistung/1 -> Gain/1
  Gain/1 -> Lagerverlustleistung/1

== system Library_ASK/Lagerverluste 2 ==
  n : Inport
  D [m] : Constant  Value=0.022
  F [N] : Constant  Value=3700
  Product : Product  Inputs=*****
  mu : Constant  Value=0.05
  pi : Constant  Value=pi
  "rad/s -> U/s" : Gain
  Out1 : Outport
  wires:
  Product/1 -> Out1/1
  n/1 -> "rad/s -> U/s"/1
  "rad/s -> U/s"/1 -> Product/5
  D [m]/1 -> Product/4
  F [N]/1 -> Product/3
  pi/1 -> Product/2
  mu/1 -> Product/1

== system Library_ASK/Leerlaufverlustgrad Verzahnung ==
  Drehzahl Ritzel : Inport
  Teilkreisdurchmesser : Inport  Port=2
  Abs : Abs
  Gain : Gain  Gain=1/20
  Product1 : Product
  Teilkreisradius : Gain  Gain=0.5
  "mm -> m" : Gain  Gain=0.001
  Leerlaufverlustgrad : Outport
  wires:
  Teilkreisdurchmesser/1 -> Teilkreisradius/1
  Teilkreisradius/1 -> "mm -> m"/1
  Drehzahl Ritzel/1 -> Abs/1
  "mm -> m"/1 -> Product1/2
  Abs/1 -> Product1/1
  Product1/1 -> Gain/1  "vt in m/s"
  Gain/1 -> Leerlaufverlustgrad/1

== system Library_ASK/Leistungselektronik ==
  note: Verlustleistungsberechnung
  Leistung : Inport
  RMS Spannung : Inport  Port=2
  Drehmoment : Inport  Port=3
  "Drehzahl " : Inport  Port=4
  Enable : EnablePort
  Abs2 : Abs
  Abs4 : Abs
  Abs5 : Abs
  Constant : Constant
  Math Function : Math  Operator=pow  SaturateOnIntegerOverflow=on
  MinMax1 : MinMax  Function=max  Inputs=2
  Powerfactorberechnung : Subsystem
  Product : Product
  Product1 : Product
  Product2 : Product
  Sign : Signum
  Stromberechnung : Subsystem
  Subtract : Sum  Inputs=+-
  "W -> kW1" : Gain  Gain=-1
  Wirkungsgradberechnung : Subsystem
  Wirkungsgrad_LE : Outport
  Verlustleistung_LE : Outport  Port=2
  Leistung_LE_DC : Outport  Port=3
  wires:
  Powerfactorberechnung/1(Powerfactor) -> Stromberechnung/3(Powerfactor), Wirkungsgradberechnung/3(Powerfactor)
  Sign/1 -> "W -> kW1"/1
  Product2/1 -> Leistung_LE_DC/1
  Wirkungsgradberechnung/1(Wirkungsgrad_LE) -> Wirkungsgrad_LE/1, Subtract/2, Math Function/1
  Abs5/1 -> Powerfactorberechnung/2(Drehzahl)
  Abs4/1 -> Powerfactorberechnung/1(Drehmoment)
  Product/1 -> MinMax1/1
  Leistung/1 -> Abs2/1, Product2/1, Sign/1
  Stromberechnung/1(Strom) -> Wirkungsgradberechnung/1(Strom)
  Math Function/1 -> Product2/2, Product/2
  "W -> kW1"/1 -> Math Function/2
  Product1/1 -> Verlustleistung_LE/1
  Subtract/1 -> Product1/2
  Constant/1 -> Subtract/1
  "Drehzahl "/1 -> Abs5/1
  RMS Spannung/1 -> Wirkungsgradberechnung/2(Spannung), Stromberechnung/2(Spannung)
  Abs2/1 -> Stromberechnung/1(Leistung), MinMax1/2, Product/1
  MinMax1/1 -> Product1/1
  Drehmoment/1 -> Abs4/1

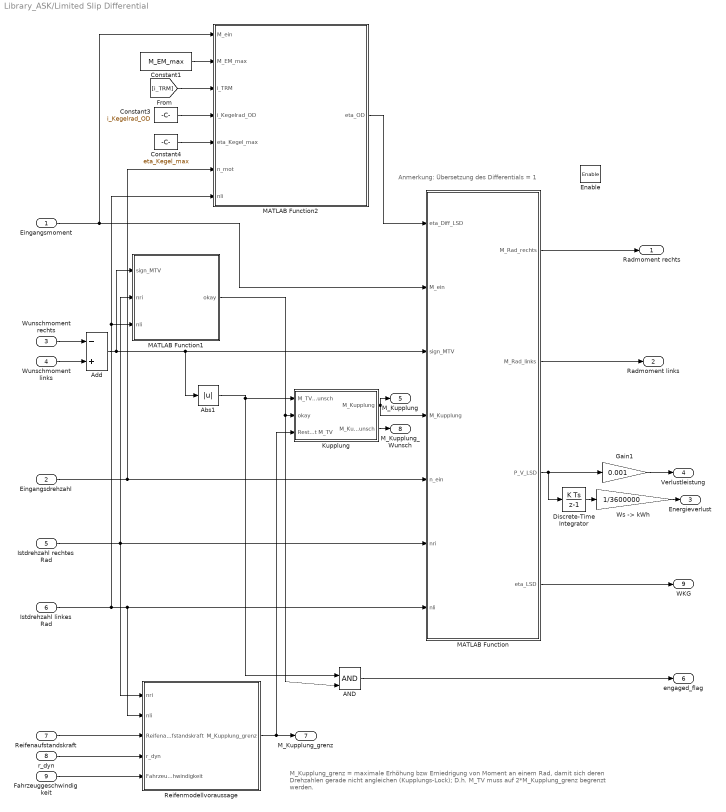
== system Library_ASK/Limited Slip Differential ==
  note: M_Kupplung_grenz = maximale Erhöhung bzw Erniedrigung von Moment an einem Rad, damit sich deren Drehzahlen
      | gerade nicht angleichen (Kupplungs-Lock);
      |
      | D.h. M_TV muss auf 2*M_Kupplung_grenz begrenzt werden.
  note: Anmerkung: Übersetzung des Differentials = 1
  Eingangsmoment : Inport
  Eingangsdrehzahl : Inport  Port=2
  Wunschmoment rechts : Inport  Port=3
  Wunschmoment links : Inport  Port=4
  Istdrehzahl rechtes Rad : Inport  Port=5
  Istdrehzahl linkes Rad : Inport  Port=6
  Reifenaufstandskraft : Inport  Port=7
  r_dyn : Inport  Port=8
  Fahrzeuggeschwindigkeit : Inport  Port=9
  Enable : EnablePort
  AND : Logic  IconShape=distinctive  AllPortsSameDT=off  OutDataTypeStr=boolean
  Abs1 : Abs
  Add : Sum  Inputs=-+
  Constant1 : Constant  Value=M_EM_max
  Constant3 : Constant  Value=i_Kegelrad_OD
  Constant4 : Constant  Value=eta_Kegel_max
  Discrete-Time Integrator : DiscreteIntegrator  gainval=1  SampleTime=-1  ICPrevOutput=DiscIntNeverNeededParam  ICPrevScaledInput=DiscIntNeverNeededParam
  Gain1 : Gain  Gain=0.001
  Kupplung : Subsystem
  MATLAB Function : MATLAB Function  TreatAsAtomicUnit=on
  MATLAB Function1 : MATLAB Function  TreatAsAtomicUnit=on
  MATLAB Function2 : MATLAB Function  TreatAsAtomicUnit=on
  Reifenmodellvoraussage : Subsystem
  "Ws -> kWh" : Gain  Gain=1/3600000
  "Radmoment rechts " : Outport  InitialOutput=0
  Radmoment links : Outport  Port=2  InitialOutput=0
  Energieverlust : Outport  Port=3  InitialOutput=0
  Verlustleistung : Outport  Port=4
  M_Kupplung : Outport  Port=5
  engaged_flag : Outport  Port=6
  M_Kupplung_grenz : Outport  Port=7
  M_Kupplung_Wunsch : Outport  Port=8
  WKG : Outport  Port=9
  wires:
  Eingangsmoment/1 -> MATLAB Function2/1(M_ein), MATLAB Function/2(M_ein)
  Eingangsdrehzahl/1 -> MATLAB Function2/6(n_mot), MATLAB Function/5(n_ein)
  Discrete-Time Integrator/1 -> "Ws -> kWh"/1
  "Ws -> kWh"/1 -> Energieverlust/1
  Istdrehzahl rechtes Rad/1 -> MATLAB Function1/2(nri), MATLAB Function/6(nri), Reifenmodellvoraussage/1(nri)
  Istdrehzahl linkes Rad/1 -> MATLAB Function/7(nli), Reifenmodellvoraussage/2(nli), MATLAB Function2/7(nli), MATLAB Function1/3(nli)
  MATLAB Function/1(M_Rad_rechts) -> "Radmoment rechts "/1
  MATLAB Function/2(M_Rad_links) -> Radmoment links/1
  MATLAB Function/3(P_V_LSD) -> Discrete-Time Integrator/1, Gain1/1
  Wunschmoment rechts/1 -> Add/1
  Wunschmoment links/1 -> Add/2
  Add/1 -> MATLAB Function/3(sign_MTV), Abs1/1, MATLAB Function1/1(sign_MTV)
  Abs1/1 -> AND/1, Kupplung/1(M_TV_Wunsch)
  Gain1/1 -> Verlustleistung/1
  Kupplung/1(M_Kupplung) -> MATLAB Function/4(M_Kupplung), M_Kupplung/1
  MATLAB Function1/1(okay) -> AND/2, Kupplung/2(okay)
  Reifenaufstandskraft/1 -> Reifenmodellvoraussage/3(Reifenaufstandskraft)
  r_dyn/1 -> Reifenmodellvoraussage/4(r_dyn)
  Fahrzeuggeschwindigkeit/1 -> Reifenmodellvoraussage/5(Fahrzeuggeschwindigkeit)
  Reifenmodellvoraussage/1(M_Kupplung_grenz) -> M_Kupplung_grenz/1, Kupplung/3(Restrict M_TV)
  AND/1 -> engaged_flag/1
  Kupplung/2(M_Kuppl_Wunsch) -> M_Kupplung_Wunsch/1
  MATLAB Function/4(eta_LSD) -> WKG/1
  [i_TRM] -> MATLAB Function2/3(i_TRM)
  Constant1/1 -> MATLAB Function2/2(M_EM_max)
  Constant3/1 -> MATLAB Function2/4(i_Kegelrad_OD)
  Constant4/1 -> MATLAB Function2/5(eta_Kegel_max)
  MATLAB Function2/1(eta_OD) -> MATLAB Function/1(eta_Diff_LSD)

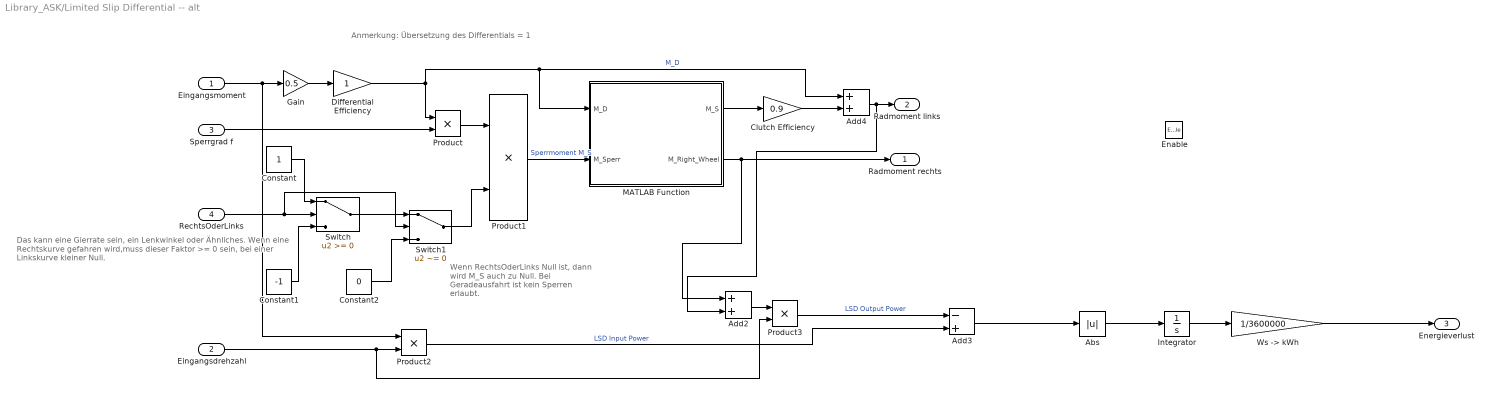
== system Library_ASK/Limited Slip Differential -- alt ==
  note: Das kann eine Gierrate sein, ein Lenkwinkel oder Ähnliches.
      | Wenn eine Rechtskurve gefahren wird,muss dieser Faktor >= 0 sein,
      | bei einer Linkskurve kleiner Null.
  note: Wenn RechtsOderLinks Null ist,
      | dann wird M_S auch zu Null.
      | Bei Geradeausfahrt ist kein Sperren
      | erlaubt.
  note: Anmerkung: Übersetzung des Differentials = 1
  Eingangsmoment : Inport
  Eingangsdrehzahl : Inport  Port=2
  Sperrgrad f : Inport  Port=3
  RechtsOderLinks : Inport  Port=4
  Enable : EnablePort
  Abs : Abs
  Add2 : Sum
  Add3 : Sum  Inputs=-+
  Add4 : Sum
  Clutch Efficiency : Gain  Gain=0.9
  Constant : Constant
  Constant1 : Constant  Value=-1
  Constant2 : Constant  Value=0
  Differential Efficiency : Gain
  Gain : Gain  Gain=0.5
  Integrator : Integrator
  MATLAB Function : Subsystem  TreatAsAtomicUnit=on
  Product{,1..3} (4 alike) : Product
  Switch : Switch  OutMin=[-1]  OutMax=[1]
  Switch1 : Switch  Criteria=u2 ~= 0  OutMin=[-1]  OutMax=[1]
  "Ws -> kWh" : Gain  Gain=1/3600000
  "Radmoment rechts " : Outport  InitialOutput=0
  Radmoment links : Outport  Port=2  InitialOutput=0
  Energieverlust : Outport  Port=3  InitialOutput=0
  wires:
  Abs/1 -> Integrator/1
  "Ws -> kWh"/1 -> Energieverlust/1
  Integrator/1 -> "Ws -> kWh"/1
  Add3/1 -> Abs/1
  Add4/1 -> Radmoment links/1, Add2/2
  MATLAB Function/2(M_Right_Wheel) -> "Radmoment rechts "/1, Add2/1
  Clutch Efficiency/1 -> Add4/2
  MATLAB Function/1(M_S) -> Clutch Efficiency/1
  Product2/1 -> Add3/2  "LSD Input Power"
  Product3/1 -> Add3/1  "LSD Output Power"
  Add2/1 -> Product3/1
  Switch1/1 -> Product1/2
  Constant2/1 -> Switch1/3
  Switch/1 -> Switch1/1
  Eingangsdrehzahl/1 -> Product2/2, Product3/2
  Differential Efficiency/1 -> MATLAB Function/1(M_D), Add4/1, Product/1  "M_D"
  Product1/1 -> MATLAB Function/2(M_Sperr)  "Sperrmoment M_S"
  Product/1 -> Product1/1
  RechtsOderLinks/1 -> Switch/2, Switch1/2
  Constant/1 -> Switch/1
  Constant1/1 -> Switch/3
  Sperrgrad f/1 -> Product/2
  Gain/1 -> Differential Efficiency/1
  Eingangsmoment/1 -> Gain/1, Product2/1

== system Library_ASK/Mehrstufiges Getriebe HA ==
  note: Lastanteil
  Eingangsmoment : Inport
  Eingangsdrehzahl : Inport  Port=2
  Enable : EnablePort
  Abs3 : Abs
  Constant1 : Constant  Value=M_EM_max
  Divide : Product  Inputs=*/
  Lastanteil : Product  Inputs=*/
  Product : Product  Inputs=3
  Product1 : Product
  Product4 : Product
  Stufenanzahl : Constant  Value=n_Stufen_TRM_HA
  Stufenübersetzung 1 : Constant  Value=i_TRM_Stufe_1_HA
  Stufenübersetzung 2 : Constant  Value=i_TRM_Stufe_2_HA
  Subsystem : Subsystem
  Terminator : Terminator
  WKG : Subsystem
  Ausgangsmoment : Outport  InitialOutput=0
  Energieverlust : Outport  Port=2  InitialOutput=0
  Verlustleistung : Outport  Port=3
  eta_GTR : Outport  Port=4
  wires:
  Stufenübersetzung 2/1 -> WKG/5(Stufenübersetzung2), Product1/2
  Subsystem/2(Verlustleistung [kW]) -> Verlustleistung/1
  Subsystem/1(Energieverlust [kWh]) -> Energieverlust/1
  Product4/1 -> Subsystem/2(Inputleistung)  "Electric Motor Input Power [W]"
  Abs3/1 -> WKG/4(Last)
  Constant1/1 -> Lastanteil/2
  Lastanteil/1 -> Abs3/1
  Stufenanzahl/1 -> WKG/2(Stufenanzahl)
  Stufenübersetzung 1/1 -> Product1/1, WKG/1(Stufenübersetzung)
  Product/1 -> Ausgangsmoment/1
  Eingangsdrehzahl/1 -> Divide/1, Product4/2, WKG/3(Eingangsdrehzahl)
  Eingangsmoment/1 -> Lastanteil/1, Product/1, Product4/1
  WKG/1(WKG) -> eta_GTR/1, Product/3, Subsystem/1(WKG)  "RF"
  Product1/1 -> Divide/2, Product/2
  Divide/1 -> Terminator/1

== system Library_ASK/Mehrstufiges Getriebe VA ==
  note: Lastanteil
  Eingangsmoment : Inport
  Eingangsdrehzahl : Inport  Port=2
  Enable : EnablePort
  Abs3 : Abs
  Constant1 : Constant  Value=M_EM_max
  Divide : Product  Inputs=*/
  Lastanteil : Product  Inputs=*/
  Product : Product  Inputs=3
  Product1 : Product
  Product4 : Product
  Scope : Scope
  Stufenanzahl : Constant  Value=n_Stufen_TRM_VA
  Stufenübersetzung 1 : Constant  Value=i_TRM_Stufe_1_VA
  Stufenübersetzung 2 : Constant  Value=i_TRM_Stufe_2_VA
  Subsystem : Subsystem
  Terminator : Terminator
  WKG : Subsystem
  Ausgangsmoment : Outport  InitialOutput=0
  Energieverlust : Outport  Port=2  InitialOutput=0
  Verlustleistung : Outport  Port=3
  eta_GTR : Outport  Port=4
  wires:
  Divide/1 -> Terminator/1
  Product1/1 -> Divide/2, Product/2
  WKG/1(WKG Pesce) -> Subsystem/1(WKG), Product/3, eta_GTR/1  "RF"
  Eingangsmoment/1 -> Product4/1, Product/1, WKG/6(Eingangsmoment), Lastanteil/1
  Eingangsdrehzahl/1 -> WKG/3(Eingangsdrehzahl), Product4/2, Divide/1
  Product/1 -> Ausgangsmoment/1
  Stufenübersetzung 1/1 -> WKG/1(Stufenübersetzung 1), Product1/1
  Stufenanzahl/1 -> WKG/2(Stufenanzahl)
  Lastanteil/1 -> Abs3/1
  Constant1/1 -> Lastanteil/2
  Abs3/1 -> WKG/4(Last)
  Product4/1 -> Subsystem/2(Inputleistung)  "Electric Motor Input Power [W]"
  Subsystem/1(Energieverlust [kWh]) -> Energieverlust/1
  Subsystem/2(Verlustleistung [kW]) -> Verlustleistung/1
  Stufenübersetzung 2/1 -> WKG/5(Stufenübersetzung 2), Product1/2
  WKG/2(WKG NWH) -> Scope/1

== system Library_ASK/Mehrstufiges und mehrgängiges Getriebe ==
  Eingangsmoment : Inport
  Eingangsdrehzahl : Inport  Port=2
  i_Gang_ges : Inport  Port=3
  WKG_max_Gang : Inport  Port=4
  Rekuperationsindex : Inport  Port=5
  Enable : EnablePort
  Math Function1 : Math  Operator=pow  SaturateOnIntegerOverflow=on
  Product : Product  Inputs=3
  Product4 : Product
  Subsystem : Subsystem
  Ausgangsmoment : Outport  InitialOutput=0
  Verlustleistung : Outport  Port=2
  eta_GTR : Outport  Port=3
  wires:
  Subsystem/1(Verlustleistung [kW]) -> Verlustleistung/1
  Product4/1 -> Subsystem/2(Inputleistung)  "Electric Motor Input Power [W]"
  Product/1 -> Ausgangsmoment/1
  Eingangsdrehzahl/1 -> Product4/2
  Eingangsmoment/1 -> Product4/1, Product/1
  i_Gang_ges/1 -> Product/2
  Rekuperationsindex/1 -> Math Function1/2
  WKG_max_Gang/1 -> eta_GTR/1, Math Function1/1, Subsystem/1(WKG)
  Math Function1/1 -> Product/3

== system Library_ASK/Momentenrückführung az HA ==
  M_Wheel_desired : Inport
  Raddrehzahl : Inport  Port=2
  eta_HA : Inport  Port=3
  Add : Sum
  Constant : Constant  Value=akt_GTR_az_HA
  Constant1 : Constant  Value=akt_2GTR_az_HA
  Demux : Demux  Outputs=2
  Fall Eingängiges Getriebe : Subsystem
  Fall zweigängiges Getriebe : Subsystem
  Gain : Gain  Gain=0.5
  Switch : Switch  Criteria=u2 > Threshold
  M_EM : Outport
  wires:
  Constant1/1 -> Fall zweigängiges Getriebe/Enable
  Constant/1 -> Fall Eingängiges Getriebe/Enable, Switch/2
  Fall zweigängiges Getriebe/1(Motorwunschmoment) -> Switch/3
  Switch/1 -> M_EM/1
  Fall Eingängiges Getriebe/1(Motorwunschmoment) -> Switch/1
  M_Wheel_desired/1 -> Fall Eingängiges Getriebe/1(Radwunschmoment), Fall zweigängiges Getriebe/1(Radwunschmoment)
  Add/1 -> Gain/1
  Demux/2 -> Add/2
  Demux/1 -> Add/1
  Raddrehzahl/1 -> Demux/1
  Gain/1 -> Fall zweigängiges Getriebe/2(Mittlere Raddrehzahl)
  eta_HA/1 -> Fall zweigängiges Getriebe/3(eta_HA), Fall Eingängiges Getriebe/2(eta_HA)

== system Library_ASK/Momentenrückführung az VA ==
  M_Wheel_desired : Inport
  Raddrehzahl : Inport  Port=2
  eta_VA : Inport  Port=3
  Add : Sum
  Constant : Constant  Value=akt_GTR_az_VA
  Constant1 : Constant  Value=akt_2GTR_az_VA
  Demux : Demux  Outputs=2
  Fall Eingängiges Getriebe : Subsystem
  Fall zweigängiges Getriebe : Subsystem
  Gain : Gain  Gain=0.5
  Switch : Switch  Criteria=u2 > Threshold
  M_EM : Outport
  wires:
  M_Wheel_desired/1 -> Fall zweigängiges Getriebe/1(Radwunschmoment), Fall Eingängiges Getriebe/1(Radwunschmoment)
  Fall Eingängiges Getriebe/1(Motorwunschmoment) -> Switch/1
  Switch/1 -> M_EM/1
  Fall zweigängiges Getriebe/1(Motorwunschmoment) -> Switch/3
  Constant/1 -> Switch/2, Fall Eingängiges Getriebe/Enable
  Constant1/1 -> Fall zweigängiges Getriebe/Enable
  Add/1 -> Gain/1
  Demux/2 -> Add/2
  Demux/1 -> Add/1
  Raddrehzahl/1 -> Demux/1
  Gain/1 -> Fall zweigängiges Getriebe/2(Mittlere Raddrehzahl)
  eta_VA/1 -> Fall zweigängiges Getriebe/3(eta_VA), Fall Eingängiges Getriebe/2(eta_VA)

== system Library_ASK/Momentenrückführung fuer mmG ==
  Radwunschmoment : Inport
  eta_VA : Inport  Port=2
  i_Gang : Inport  Port=3
  Rekuperationsindex : Inport  Port=4
  Enable : EnablePort
  Divide1 : Product  Inputs=*//
  Math Function : Math  Operator=pow  SaturateOnIntegerOverflow=on
  M_EM : Outport
  wires:
  i_Gang/1 -> Divide1/2
  eta_VA/1 -> Math Function/1
  Radwunschmoment/1 -> Divide1/1
  Divide1/1 -> M_EM/1
  Rekuperationsindex/1 -> Math Function/2
  Math Function/1 -> Divide1/3

== system Library_ASK/Momentenrückführung rn HA ==
  M_Wheel_desired : Inport
  Raddrehzahl : Inport  Port=2
  eta_HA : Inport  Port=3
  Constant : Constant  Value=akt_GTR_rn_HA
  Constant1 : Constant  Value=akt_2GTR_rn_HA
  Fall Eingängiges Getriebe : Subsystem
  Fall zweigängiges Getriebe : Subsystem
  Switch : Switch  Criteria=u2 > Threshold
  M_EM : Outport
  wires:
  Raddrehzahl/1 -> Fall zweigängiges Getriebe/2(Raddrehzahl)
  M_Wheel_desired/1 -> Fall zweigängiges Getriebe/1(Radwunschmoment), Fall Eingängiges Getriebe/1(Radwunschmoment)
  Fall Eingängiges Getriebe/1(Motorwunschmoment) -> Switch/1
  Switch/1 -> M_EM/1
  Fall zweigängiges Getriebe/1(Motorwunschmoment) -> Switch/3
  Constant/1 -> Switch/2, Fall Eingängiges Getriebe/Enable
  Constant1/1 -> Fall zweigängiges Getriebe/Enable
  eta_HA/1 -> Fall zweigängiges Getriebe/3(eta_HA), Fall Eingängiges Getriebe/2(eta_HA)

== system Library_ASK/Momentenrückführung rn VA ==
  M_Wheel_desired : Inport
  Raddrehzahl : Inport  Port=2
  eta_VA : Inport  Port=3
  Constant : Constant  Value=akt_GTR_rn_VA
  Constant1 : Constant  Value=akt_2GTR_rn_VA
  Fall Eingängiges Getriebe : Subsystem
  Fall zweigängiges Getriebe : Subsystem
  Switch : Switch  Criteria=u2 > Threshold
  M_EM : Outport
  wires:
  Constant1/1 -> Fall zweigängiges Getriebe/Enable
  Constant/1 -> Fall Eingängiges Getriebe/Enable, Switch/2
  Fall zweigängiges Getriebe/1(Motorwunschmoment) -> Switch/3
  Switch/1 -> M_EM/1
  Fall Eingängiges Getriebe/1(Motorwunschmoment) -> Switch/1
  M_Wheel_desired/1 -> Fall Eingängiges Getriebe/1(Radwunschmoment), Fall zweigängiges Getriebe/1(Radwunschmoment)
  Raddrehzahl/1 -> Fall zweigängiges Getriebe/2(Raddrehzahl)
  eta_VA/1 -> Fall zweigängiges Getriebe/3(eta_VA), Fall Eingängiges Getriebe/2(eta_VA)

== system Library_ASK/NWH Planetengetriebe ==
  note: Umfangskraft Planententeilkreis
  note: Grundkreisdurchmesser in Geometrieberechnung berechenbar (aus Größen, die innerhalb einer Simulation feststehen).
      | Drehzahl Ritzel muss rückgeführt werden aus der eUELG - Hauptfunktion, ebenfalls das Moment des Steges.
      | Das Drehmoment am Steg ergibt dann über die Geometrie die Umfangskraft am Planeten im Teilkreis.
  Standübersetzung der Stufe : Inport
  Drehzahl Planet : Inport  Port=2
  Stegmoment : Inport  Port=3
  Durchmesser Steg : Inport  Port=4
  Teilkreis Planet : Inport  Port=5
  z_Rad : Inport  Port=6
  Abs : Abs
  Abs1 : Abs
  Add : Sum  Inputs=+-
  Berechnung Hv : Subsystem
  Berechnung mu : Subsystem
  Constant : Constant
  Divide : Product  Inputs=/*
  Divide1 : Product  Inputs=*/
  Eingriffswinkel : Constant  Value=alpha
  Gain : Gain  Gain=0.5
  "Nm -> Nmm" : Gain  Gain=1000
  Product : Product
  "Teilkreis -> Grundkreis" : Product  Inputs=*/
  Trigonometric Function : Trigonometry  Operator=cos
  Verzahnungswirkungsgrad aus Last : Outport
  mu : Outport  Port=2
  wires:
  Berechnung Hv/1(Hv) -> Product/2
  Berechnung mu/1(mu) -> mu/1, Product/1
  z_Rad/1 -> Divide/2, Berechnung Hv/2(z_Rad)
  Divide/1 -> Berechnung Hv/1(z_Ritzel)
  Standübersetzung der Stufe/1 -> Divide/1
  Drehzahl Planet/1 -> Abs/1
  Stegmoment/1 -> "Nm -> Nmm"/1
  Durchmesser Steg/1 -> Divide1/2
  Divide1/1 -> Gain/1
  "Teilkreis -> Grundkreis"/1 -> Abs1/1
  Trigonometric Function/1 -> "Teilkreis -> Grundkreis"/2
  Eingriffswinkel/1 -> Trigonometric Function/1
  Product/1 -> Add/2
  Constant/1 -> Add/1
  Add/1 -> Verzahnungswirkungsgrad aus Last/1
  Teilkreis Planet/1 -> Berechnung mu/3(Teilkreisdurchmesser)
  Gain/1 -> "Teilkreis -> Grundkreis"/1
  "Nm -> Nmm"/1 -> Divide1/1
  Abs/1 -> Berechnung mu/2(Drehzahl Planet)
  Abs1/1 -> Berechnung mu/1(Umfangskraft am Grundkreis)

== system Library_ASK/NWH Stufengetriebe ==
  note: Umfangskraft Ritzelteilkreis
  Standübersetzung der Stufe : Inport
  Drehzahl Ritzel : Inport  Port=2
  Moment Ritzel : Inport  Port=3
  Teilkreisdurchmesser Ritzel : Inport  Port=4
  z_Rad : Inport  Port=5
  Teilkreisdurchmesser Rad : Inport  Port=6
  Abs : Abs
  Abs1 : Abs
  Add : Sum  Inputs=+-
  Berechnung Hv : Subsystem
  Berechnung mu : Subsystem
  Constant : Constant
  Divide : Product  Inputs=/*
  Divide1 : Product  Inputs=*/
  Eingriffswinkel : Constant  Value=alpha
  Gain : Gain  Gain=0.5
  "Nm -> Nmm" : Gain  Gain=1000
  Product : Product
  "Teilkreis -> Grundkreis" : Product  Inputs=*/
  Trigonometric Function : Trigonometry  Operator=cos
  Verzahnungswirkungsgrad aus Last : Outport
  mu : Outport  Port=2
  wires:
  Abs1/1 -> Berechnung mu/1(Umfangskraft am Grundkreis)
  Abs/1 -> Berechnung mu/2(Drehzahl Planet)
  "Nm -> Nmm"/1 -> Divide1/1
  Gain/1 -> "Teilkreis -> Grundkreis"/1
  Teilkreisdurchmesser Ritzel/1 -> Divide1/2, Berechnung mu/3(Teilkreisdurchmesser Ritzel)
  Add/1 -> Verzahnungswirkungsgrad aus Last/1
  Constant/1 -> Add/1
  Product/1 -> Add/2
  Eingriffswinkel/1 -> Trigonometric Function/1
  Trigonometric Function/1 -> "Teilkreis -> Grundkreis"/2
  "Teilkreis -> Grundkreis"/1 -> Abs1/1
  Divide1/1 -> Gain/1
  Moment Ritzel/1 -> "Nm -> Nmm"/1
  Drehzahl Ritzel/1 -> Abs/1
  Standübersetzung der Stufe/1 -> Divide/1
  Divide/1 -> Berechnung Hv/1(z_Ritzel)
  z_Rad/1 -> Berechnung Hv/2(z_Rad), Divide/2
  Berechnung mu/1(mu) -> mu/1, Product/1
  Berechnung Hv/1(Hv) -> Product/2
  Teilkreisdurchmesser Rad/1 -> Berechnung mu/4(Teilkreisdurchmesser Rad)

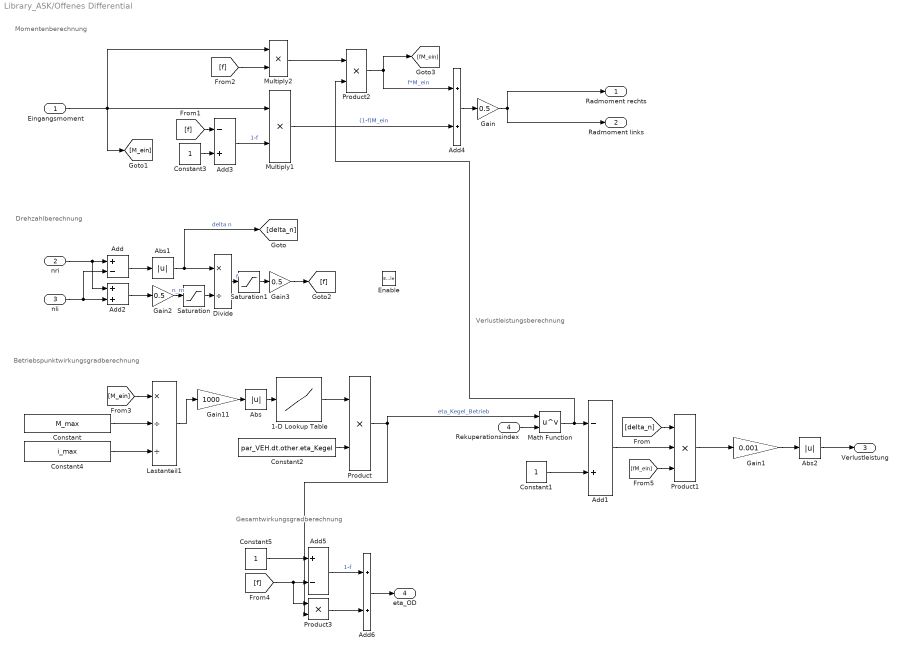
== system Library_ASK/Offenes Differential ==
  note: Gesamtwirkungsgradberechnung
  note: Momentenberechnung
  note: Verlustleistungsberechnung
  note: Drehzahlberechnung
  note: Betriebspunktwirkungsgradberechnung
  Eingangsmoment : Inport
  nri : Inport  Port=2
  nli : Inport  Port=3
  Rekuperationsindex : Inport  Port=4
  Enable : EnablePort
  1-D Lookup Table : Lookup_n-D  NumberOfTableDimensions=1  BreakpointsForDimension1=par_VEH.dt.other.wkg_last_bp  Table=par_VEH.dt.other.wkg_last  ExtrapMethod=Clip  InternalRulePriority=Speed  RndMeth=Simplest  InputSameDT=on
  Abs : Abs
  Abs1 : Abs
  Abs2 : Abs
  Add : Sum  Inputs=+-
  Add1 : Sum  Inputs=-+
  Add2 : Sum
  Add3 : Sum  Inputs=-+
  Add4 : Sum
  Add5 : Sum  Inputs=+-
  Add6 : Sum
  Constant : Constant  Value=M_max
  Constant1 : Constant
  Constant2 : Constant  Value=par_VEH.dt.other.eta_Kegel
  Constant3 : Constant
  Constant4 : Constant  Value=i_max
  Constant5 : Constant
  Divide : Product  Inputs=*/
  Gain : Gain  Gain=0.5
  Gain1 : Gain  Gain=0.001
  Gain11 : Gain  Gain=1000
  Gain2 : Gain  Gain=0.5
  Gain3 : Gain  Gain=0.5
  Lastanteil1 : Product  Inputs=*//
  Math Function : Math  Operator=pow  SaturateOnIntegerOverflow=on
  Multiply1 : Product  Inputs=**
  Multiply2 : Product  Inputs=**
  Product : Product
  Product1 : Product  Inputs=3
  Product2 : Product
  Product3 : Product
  Saturation : Saturate  UpperLimit=inf  LowerLimit=0.01
  Saturation1 : Saturate  UpperLimit=1  LowerLimit=0
  Radmoment rechts : Outport  InitialOutput=0
  Radmoment links : Outport  Port=2
  Verlustleistung : Outport  Port=3
  eta_OD : Outport  Port=4
  wires:
  Add1/1 -> Product1/2
  Product1/1 -> Gain1/1
  Constant1/1 -> Add1/2
  Constant2/1 -> Product/2
  1-D Lookup Table/1 -> Product/1
  Add/1 -> Abs1/1
  nli/1 -> Add2/2, Add/2
  nri/1 -> Add2/1, Add/1
  Abs/1 -> 1-D Lookup Table/1
  Rekuperationsindex/1 -> Math Function/2
  Product/1 -> Math Function/1, Product3/2  "eta_Kegel_Betrieb"
  Math Function/1 -> Add1/1, Product2/2
  Eingangsmoment/1 -> [M_ein], Multiply2/1, Multiply1/1
  Gain/1 -> Radmoment rechts/1, Radmoment links/1
  Gain1/1 -> Abs2/1
  Constant/1 -> Lastanteil1/2
  Constant4/1 -> Lastanteil1/3
  Gain11/1 -> Abs/1
  Lastanteil1/1 -> Gain11/1
  Abs1/1 -> [delta_n], Divide/1  "delta n"
  Add2/1 -> Gain2/1
  Gain2/1 -> Saturation/1  "n_m"
  Constant3/1 -> Add3/2
  Add3/1 -> Multiply1/2  "1-f"
  Multiply1/1 -> Add4/2  "(1-f)M_ein"
  Multiply2/1 -> Product2/1
  Product2/1 -> Add4/1, [fM_ein]  "f*M_ein"
  Add4/1 -> Gain/1
  [delta_n] -> Product1/1
  Divide/1 -> Saturation1/1  "f"
  [f] -> Add3/1
  [f] -> Multiply2/2
  [M_ein] -> Lastanteil1/1
  [fM_ein] -> Product1/3
  Add5/1 -> Add6/1  "1-f"
  Constant5/1 -> Add5/1
  [f] -> Product3/1, Add5/2
  Product3/1 -> Add6/2
  Add6/1 -> eta_OD/1
  Saturation/1 -> Divide/2
  Saturation1/1 -> Gain3/1
  Abs2/1 -> Verlustleistung/1
  Gain3/1 -> [f]

== system Library_ASK/Poppinga ==
  i : Inport
  z1 : Inport  Port=2
  Add : Sum  Inputs=+-
  Add1 : Sum  Inputs=+-
  Constant : Constant  Value=pi
  Constant1 : Constant
  Constant2 : Constant
  Divide : Product  Inputs=*/
  Divide1 : Product  Inputs=*****/
  Gain : Gain  Gain=2
  Zahnformfaktor : Constant
  mu : Constant  Value=0.05
  Überdeckung : Constant  Value=1.4
  eta : Outport
  wires:
  Constant1/1 -> Divide/1, Add/1
  i/1 -> Divide/2
  Divide/1 -> Add/2
  z1/1 -> Gain/1
  Add/1 -> Divide1/1
  Zahnformfaktor/1 -> Divide1/2
  mu/1 -> Divide1/3
  Constant/1 -> Divide1/4
  Überdeckung/1 -> Divide1/5
  Gain/1 -> Divide1/6
  Divide1/1 -> Add1/2
  Constant2/1 -> Add1/1
  Add1/1 -> eta/1
